simulink model "Sensor_filter_discrete_sfun"  (Simulink 7.4)
settings: Solver=FixedStepDiscrete  StartTime=0.0  StopTime=tend  FixedStep=Ts  RelTol=1e-3
values from neighbouring files (symbols this model uses):
  Ts = 0.01    [complementary_filter_param.m]    (also in quadrocopter_param.m)
settings Model: Creator=Sreekanth  LastModifiedBy=Sreekanth

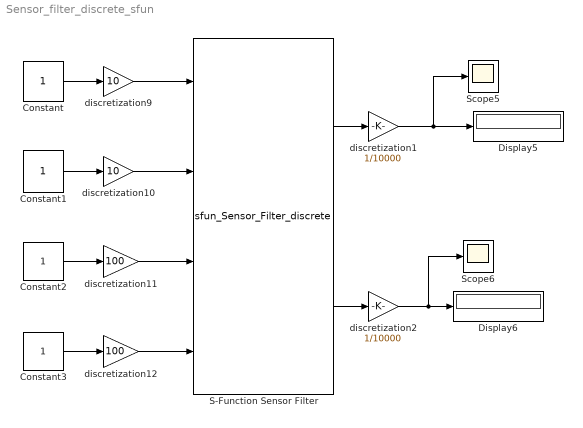
== system Sensor_filter_discrete_sfun ==
  Constant{,1..3} (4 alike) : Constant  OutDataType=fixdt(1, 16)  OutScaling=2^0  SampleTime=Ts
  Display5 : Display
  Display6 : Display
  S-Function Sensor Filter : S-Function  FunctionName=sfun_Sensor_Filter_discrete  EnableBusSupport=off
      mask Display:
      | port_label('input',1,'acc_x_B')
      | port_label('input',2,'acc_y_B')
      | port_label('input',3,'anv_phi_B')
      | port_label('input',4,'anv_theta_B')
      | port_label('output',1,'phi_filt')
      | port_label('output',2,'theta_filt')
  Scope5 : Scope
  Scope6 : Scope
  discretization1 : Gain  Gain=1/10000  ParameterDataType=fixdt(1, 16)  ParameterScaling=2^0  OutDataTypeMode=double  OutDataType=fixdt(1, 16)  OutScaling=2^0  OutDataTypeStr=double
  discretization10 : Gain  Gain=10  ParameterDataType=fixdt(1, 16)  ParameterScaling=2^0  OutDataTypeMode=int16  OutDataType=fixdt(1, 16)  OutScaling=2^0  OutDataTypeStr=int16
  discretization11 : Gain  Gain=100  ParameterDataType=fixdt(1, 16)  ParameterScaling=2^0  OutDataTypeMode=int16  OutDataType=fixdt(1, 16)  OutScaling=2^0  OutDataTypeStr=int16
  discretization12 : Gain  Gain=100  ParameterDataType=fixdt(1, 16)  ParameterScaling=2^0  OutDataTypeMode=int16  OutDataType=fixdt(1, 16)  OutScaling=2^0  OutDataTypeStr=int16
  discretization2 : Gain  Gain=1/10000  ParameterDataType=fixdt(1, 16)  ParameterScaling=2^0  OutDataTypeMode=double  OutDataType=fixdt(1, 16)  OutScaling=2^0  OutDataTypeStr=double
  discretization9 : Gain  Gain=10  ParameterDataType=fixdt(1, 16)  ParameterScaling=2^0  OutDataTypeMode=int16  OutDataType=fixdt(1, 16)  OutScaling=2^0  OutDataTypeStr=int16
  wires:
  discretization9/1 -> S-Function Sensor Filter/1
  discretization10/1 -> S-Function Sensor Filter/2
  discretization11/1 -> S-Function Sensor Filter/3
  discretization12/1 -> S-Function Sensor Filter/4
  Constant/1 -> discretization9/1
  Constant1/1 -> discretization10/1
  Constant2/1 -> discretization11/1
  Constant3/1 -> discretization12/1
  S-Function Sensor Filter/1 -> discretization1/1
  S-Function Sensor Filter/2 -> discretization2/1
  discretization1/1 -> Scope5/1, Display5/1
  discretization2/1 -> Display6/1, Scope6/1
